simulink model "Cruise_Control_system_simulation"  (R2022b)
settings: Solver=VariableStepAuto  StartTime=0.0  StopTime=100  RelTol=1e-3
undefined symbols (not defined in the file): magnitude
libraries: slpidlib x5, simulink x1
settings Model: Creator=snazari  LastModifiedBy=ayush
settings SolverCC: ZeroCrossControl=DisableAll

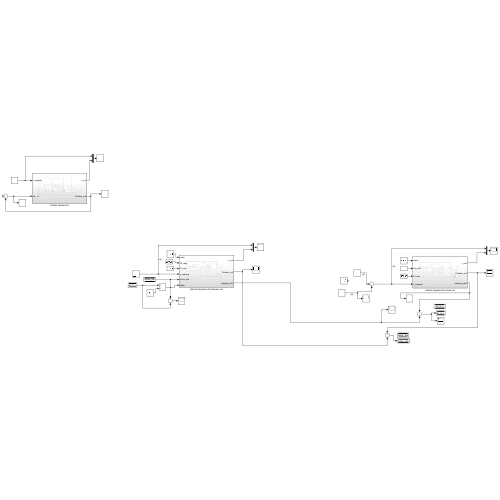
[thumbnail: Simulink's stored preview of the top-level diagram]
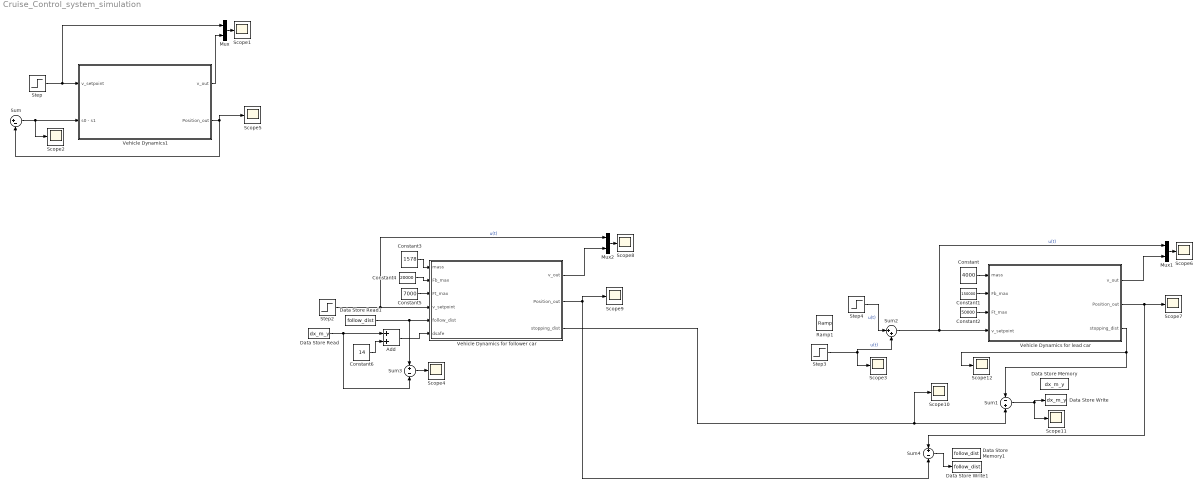
== system Cruise_Control_system_simulation ==
  Add : Sum
  Constant : Constant  Value=4000
  Constant1 : Constant  Value=150000
  Constant2 : Constant  Value=50000
  Constant3 : Constant  Value=1578
  Constant4 : Constant  Value=20000
  Constant5 : Constant  Value=7000
  Constant6 : Constant  Value=14
  Data Store Memory : DataStoreMemory  DataStoreName=dx_m_y  WriteAfterWriteMsg=warning  ShowAdditionalParam=off
  Data Store Memory1 : DataStoreMemory  DataStoreName=follow_dist  WriteAfterWriteMsg=warning  ShowAdditionalParam=off
  Data Store Read : DataStoreRead  DataStoreName=dx_m_y  IndexOptions=Index vector (dialog)  Indices=1  OutputSizes=1
  Data Store Read1 : DataStoreRead  DataStoreName=follow_dist  IndexOptions=Index vector (dialog)  Indices=1  OutputSizes=1
  Data Store Write : DataStoreWrite  DataStoreName=dx_m_y  IndexOptions=Index vector (dialog)  Indices=1  OutputSizes=1
  Data Store Write1 : DataStoreWrite  DataStoreName=follow_dist  IndexOptions=Index vector (dialog)  Indices=1  OutputSizes=1
  Mux : Mux  Inputs=2
  Mux1 : Mux  Inputs=2
  Mux2 : Mux  Inputs=2
  Ramp1 : simulink/Sources/Ramp  slope=-20  start=50  InitialOutput=0
  Scope{1..12} (12 alike) : Scope
  Step : Step  Before=3  After=35  SampleTime=0
  Step2 : Step  After=40  SampleTime=0
  Step3 : Step  Time=50  After=-35  SampleTime=0
  Step4 : Step  After=35  SampleTime=0
  Sum : Sum  Inputs=|+-
  Sum1 : Sum  Inputs=-+
  Sum2 : Sum  Inputs=|++
  Sum3 : Sum  Inputs=+-
  Sum4 : Sum  Inputs=+-
  Vehicle Dynamics for follower car : Subsystem
  Vehicle Dynamics for lead car : Subsystem
  Vehicle Dynamics1 : Subsystem
  wires:
  Constant1/1 -> Vehicle Dynamics for lead car/2(Fb_max)
  Constant/1 -> Vehicle Dynamics for lead car/1(mass)
  Sum2/1 -> Mux1/1, Vehicle Dynamics for lead car/4(v_setpoint)  "u(t)"
  Constant2/1 -> Vehicle Dynamics for lead car/3(Ft_max)
  Step3/1 -> Sum2/2, Scope3/1  "u(t)"
  Step4/1 -> Sum2/1  "u(t)"
  Mux1/1 -> Scope6/1
  Vehicle Dynamics for lead car/1(v_out) -> Mux1/2
  Vehicle Dynamics for lead car/2(Position_out) -> Sum4/1, Scope7/1
  Vehicle Dynamics for lead car/3(stopping_dist) -> Scope12/1, Sum1/1
  Step2/1 -> Mux2/1, Vehicle Dynamics for follower car/4(v_setpoint)  "u(t)"
  Mux2/1 -> Scope8/1
  Vehicle Dynamics for follower car/2(Position_out) -> Scope9/1, Sum4/2
  Constant3/1 -> Vehicle Dynamics for follower car/1(mass)
  Constant5/1 -> Vehicle Dynamics for follower car/3(Ft_max)
  Constant4/1 -> Vehicle Dynamics for follower car/2(Fb_max)
  Vehicle Dynamics for follower car/1(v_out) -> Mux2/2
  Vehicle Dynamics for follower car/3(stopping_dist) -> Scope10/1, Sum1/2
  Sum/1 -> Vehicle Dynamics1/2(s0 - s1), Scope2/1
  Vehicle Dynamics1/1(v_out) -> Mux/2
  Vehicle Dynamics1/2(Position_out) -> Scope5/1, Sum/2
  Mux/1 -> Scope1/1
  Step/1 -> Mux/1, Vehicle Dynamics1/1(v_setpoint)
  Sum4/1 -> Data Store Write1/1
  Data Store Read/1 -> Add/1, Sum3/2
  Data Store Read1/1 -> Vehicle Dynamics for follower car/5(follow_dist), Sum3/1
  Sum3/1 -> Scope4/1
  Constant6/1 -> Add/2
  Add/1 -> Vehicle Dynamics for follower car/6(dsafe)
  Sum1/1 -> Scope11/1, Data Store Write/1

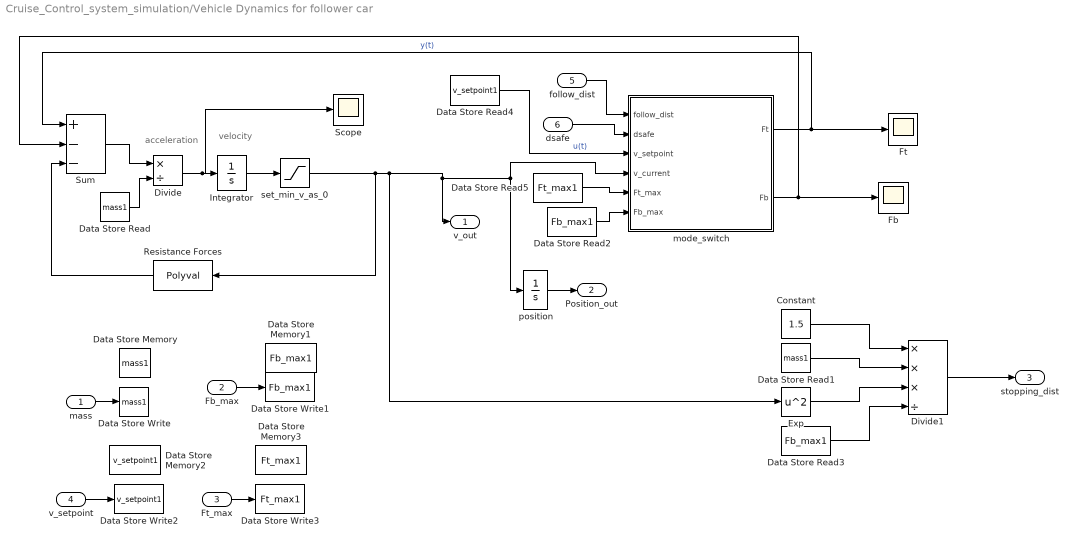
== system Cruise_Control_system_simulation/Vehicle Dynamics for follower car ==
  note: acceleration
  note: velocity
  mass : Inport
  Fb_max : Inport  Port=2
  Ft_max : Inport  Port=3
  v_setpoint : Inport  Port=4
  follow_dist : Inport  Port=5
  dsafe : Inport  Port=6
  Constant : Constant  Value=1.5
  Data Store Memory : DataStoreMemory  DataStoreName=mass1  WriteAfterWriteMsg=warning  ShowAdditionalParam=off
  Data Store Memory1 : DataStoreMemory  DataStoreName=Fb_max1  WriteAfterWriteMsg=warning  ShowAdditionalParam=off
  Data Store Memory2 : DataStoreMemory  DataStoreName=v_setpoint1  WriteAfterWriteMsg=warning  ShowAdditionalParam=off
  Data Store Memory3 : DataStoreMemory  DataStoreName=Ft_max1  WriteAfterWriteMsg=warning  ShowAdditionalParam=off
  Data Store Read : DataStoreRead  DataStoreName=mass1  IndexOptions=Index vector (dialog)  Indices=1  OutputSizes=1
  Data Store Read1 : DataStoreRead  DataStoreName=mass1  IndexOptions=Index vector (dialog)  Indices=1  OutputSizes=1
  Data Store Read2 : DataStoreRead  DataStoreName=Fb_max1  IndexOptions=Index vector (dialog)  Indices=1  OutputSizes=1
  Data Store Read3 : DataStoreRead  DataStoreName=Fb_max1  IndexOptions=Index vector (dialog)  Indices=1  OutputSizes=1
  Data Store Read4 : DataStoreRead  DataStoreName=v_setpoint1  IndexOptions=Index vector (dialog)  Indices=1  OutputSizes=1
  Data Store Read5 : DataStoreRead  DataStoreName=Ft_max1  IndexOptions=Index vector (dialog)  Indices=1  OutputSizes=1
  Data Store Write : DataStoreWrite  DataStoreName=mass1  IndexOptions=Index vector (dialog)  Indices=1  OutputSizes=1
  Data Store Write1 : DataStoreWrite  DataStoreName=Fb_max1  IndexOptions=Index vector (dialog)  Indices=1  OutputSizes=1
  Data Store Write2 : DataStoreWrite  DataStoreName=v_setpoint1  IndexOptions=Index vector (dialog)  Indices=1  OutputSizes=1
  Data Store Write3 : DataStoreWrite  DataStoreName=Ft_max1  IndexOptions=Index vector (dialog)  Indices=1  OutputSizes=1
  Divide : Product  Inputs=*/
  Divide1 : Product  Inputs=***/
  Exp : Math  Operator=square
  Fb : Scope
  Ft : Scope
  Integrator : Integrator
  Resistance Forces : Polyval  Coefs=[0.497 4.0349 97.33]
  Scope : Scope
  Sum : Sum  Inputs=+--
  mode_switch : Subsystem
  position : Integrator
  set_min_v_as_0 : Saturate  UpperLimit=3000  LowerLimit=0
  v_out : Outport
  Position_out : Outport  Port=2
  stopping_dist : Outport  Port=3
  wires:
  Data Store Read4/1 -> mode_switch/3(v_setpoint)  "u(t)"
  Integrator/1 -> set_min_v_as_0/1
  position/1 -> Position_out/1
  Resistance Forces/1 -> Sum/3
  Sum/1 -> Divide/1
  mass/1 -> Data Store Write/1
  Divide/1 -> Scope/1, Integrator/1
  mode_switch/1(Ft) -> Ft/1, Sum/1  "y(t)"
  mode_switch/2(Fb) -> Fb/1, Sum/2
  set_min_v_as_0/1 -> Exp/1, mode_switch/4(v_current), position/1, v_out/1, Resistance Forces/1
  Data Store Read5/1 -> mode_switch/5(Ft_max)
  Data Store Read2/1 -> mode_switch/6(Fb_max)
  Data Store Read/1 -> Divide/2
  Fb_max/1 -> Data Store Write1/1
  Constant/1 -> Divide1/1
  Data Store Read1/1 -> Divide1/2
  Exp/1 -> Divide1/3
  Data Store Read3/1 -> Divide1/4
  Divide1/1 -> stopping_dist/1
  v_setpoint/1 -> Data Store Write2/1
  Ft_max/1 -> Data Store Write3/1
  dsafe/1 -> mode_switch/2(dsafe)
  follow_dist/1 -> mode_switch/1(follow_dist)

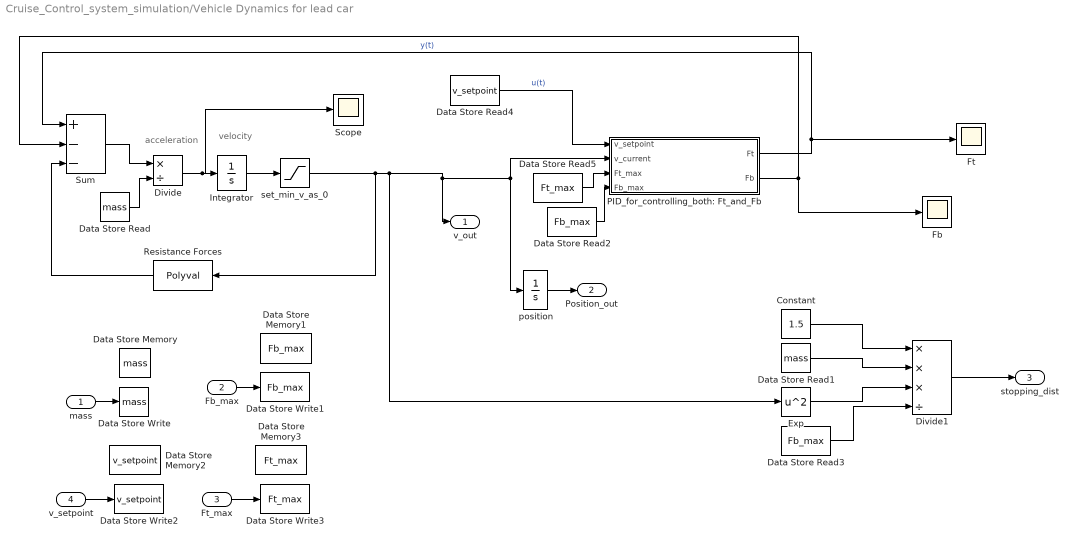
== system Cruise_Control_system_simulation/Vehicle Dynamics for lead car ==
  note: acceleration
  note: velocity
  mass : Inport
  Fb_max : Inport  Port=2
  Ft_max : Inport  Port=3
  v_setpoint : Inport  Port=4
  Constant : Constant  Value=1.5
  Data Store Memory : DataStoreMemory  DataStoreName=mass  WriteAfterWriteMsg=warning  ShowAdditionalParam=off
  Data Store Memory1 : DataStoreMemory  DataStoreName=Fb_max  WriteAfterWriteMsg=warning  ShowAdditionalParam=off
  Data Store Memory2 : DataStoreMemory  DataStoreName=v_setpoint  WriteAfterWriteMsg=warning  ShowAdditionalParam=off
  Data Store Memory3 : DataStoreMemory  DataStoreName=Ft_max  WriteAfterWriteMsg=warning  ShowAdditionalParam=off
  Data Store Read : DataStoreRead  DataStoreName=mass  IndexOptions=Index vector (dialog)  Indices=1  OutputSizes=1
  Data Store Read1 : DataStoreRead  DataStoreName=mass  IndexOptions=Index vector (dialog)  Indices=1  OutputSizes=1
  Data Store Read2 : DataStoreRead  DataStoreName=Fb_max  IndexOptions=Index vector (dialog)  Indices=1  OutputSizes=1
  Data Store Read3 : DataStoreRead  DataStoreName=Fb_max  IndexOptions=Index vector (dialog)  Indices=1  OutputSizes=1
  Data Store Read4 : DataStoreRead  DataStoreName=v_setpoint  IndexOptions=Index vector (dialog)  Indices=1  OutputSizes=1
  Data Store Read5 : DataStoreRead  DataStoreName=Ft_max  IndexOptions=Index vector (dialog)  Indices=1  OutputSizes=1
  Data Store Write : DataStoreWrite  DataStoreName=mass  IndexOptions=Index vector (dialog)  Indices=1  OutputSizes=1
  Data Store Write1 : DataStoreWrite  DataStoreName=Fb_max  IndexOptions=Index vector (dialog)  Indices=1  OutputSizes=1
  Data Store Write2 : DataStoreWrite  DataStoreName=v_setpoint  IndexOptions=Index vector (dialog)  Indices=1  OutputSizes=1
  Data Store Write3 : DataStoreWrite  DataStoreName=Ft_max  IndexOptions=Index vector (dialog)  Indices=1  OutputSizes=1
  Divide : Product  Inputs=*/
  Divide1 : Product  Inputs=***/
  Exp : Math  Operator=square
  Fb : Scope
  Ft : Scope
  Integrator : Integrator
  PID_for_controlling_both: Ft_and_Fb : Subsystem
  Resistance Forces : Polyval  Coefs=[0.497 4.0349 97.33]
  Scope : Scope
  Sum : Sum  Inputs=+--
  position : Integrator
  set_min_v_as_0 : Saturate  UpperLimit=3000  LowerLimit=0
  v_out : Outport
  Position_out : Outport  Port=2
  stopping_dist : Outport  Port=3
  wires:
  Data Store Read4/1 -> PID_for_controlling_both: Ft_and_Fb/1(v_setpoint)  "u(t)"
  Integrator/1 -> set_min_v_as_0/1
  position/1 -> Position_out/1
  Resistance Forces/1 -> Sum/3
  Sum/1 -> Divide/1
  mass/1 -> Data Store Write/1
  Divide/1 -> Scope/1, Integrator/1
  PID_for_controlling_both: Ft_and_Fb/1(Ft) -> Ft/1, Sum/1  "y(t)"
  PID_for_controlling_both: Ft_and_Fb/2(Fb) -> Fb/1, Sum/2
  set_min_v_as_0/1 -> Exp/1, PID_for_controlling_both: Ft_and_Fb/2(v_current), position/1, v_out/1, Resistance Forces/1
  Data Store Read5/1 -> PID_for_controlling_both: Ft_and_Fb/3(Ft_max)
  Data Store Read2/1 -> PID_for_controlling_both: Ft_and_Fb/4(Fb_max)
  Data Store Read/1 -> Divide/2
  Fb_max/1 -> Data Store Write1/1
  Constant/1 -> Divide1/1
  Data Store Read1/1 -> Divide1/2
  Exp/1 -> Divide1/3
  Divide1/1 -> stopping_dist/1
  v_setpoint/1 -> Data Store Write2/1
  Ft_max/1 -> Data Store Write3/1
  Data Store Read3/1 -> Divide1/4

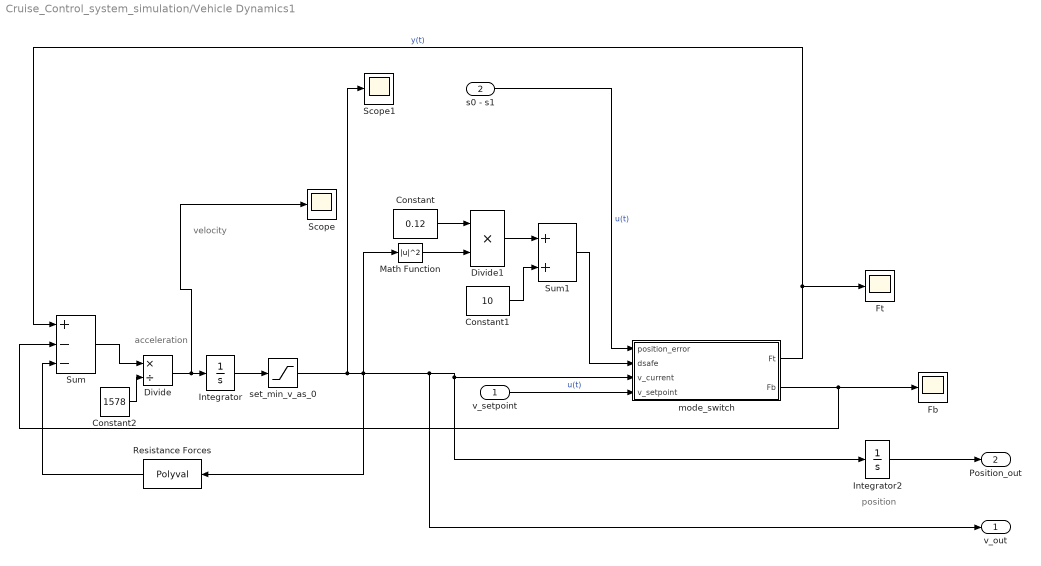
== system Cruise_Control_system_simulation/Vehicle Dynamics1 ==
  note: position
  note: acceleration
  note: velocity
  v_setpoint : Inport
  s0 - s1 : Inport  Port=2
  Constant : Constant  Value=0.12
  Constant1 : Constant  Value=10
  Constant2 : Constant  Value=1578
  Divide : Product  Inputs=*/
  Divide1 : Product  Inputs=**
  Fb : Scope
  Ft : Scope
  Integrator : Integrator
  Integrator2 : Integrator
  Math Function : Math  Operator=magnitude^2
  Resistance Forces : Polyval  Coefs=[0.497 4.0349 97.33]
  Scope : Scope
  Scope1 : Scope
  Sum : Sum  Inputs=+--
  Sum1 : Sum
  mode_switch : Subsystem
  set_min_v_as_0 : Saturate  UpperLimit=3000  LowerLimit=0
  v_out : Outport
  Position_out : Outport  Port=2
  wires:
  Divide/1 -> Scope/1, Integrator/1
  set_min_v_as_0/1 -> Math Function/1, mode_switch/3(v_current), Integrator2/1, v_out/1, Resistance Forces/1, Scope1/1
  Constant2/1 -> Divide/2
  mode_switch/2(Fb) -> Sum/2, Fb/1
  mode_switch/1(Ft) -> Sum/1, Ft/1  "y(t)"
  Resistance Forces/1 -> Sum/3
  Integrator2/1 -> Position_out/1
  Sum/1 -> Divide/1
  Integrator/1 -> set_min_v_as_0/1
  s0 - s1/1 -> mode_switch/1(position_error)  "u(t)"
  v_setpoint/1 -> mode_switch/4(v_setpoint)  "u(t)"
  Constant/1 -> Divide1/1
  Math Function/1 -> Divide1/2
  Divide1/1 -> Sum1/1
  Sum1/1 -> mode_switch/2(dsafe)
  Constant1/1 -> Sum1/2

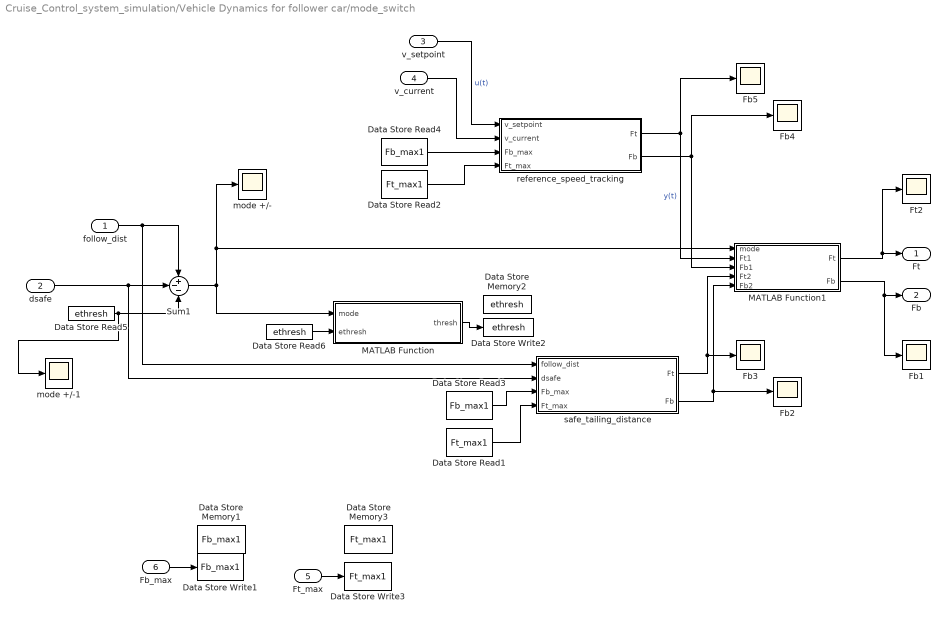
== system Cruise_Control_system_simulation/Vehicle Dynamics for follower car/mode_switch ==
  follow_dist : Inport
  dsafe : Inport  Port=2
  v_setpoint : Inport  Port=3
  v_current : Inport  Port=4
  Ft_max : Inport  Port=5
  Fb_max : Inport  Port=6
  Data Store Memory1 : DataStoreMemory  DataStoreName=Fb_max1  WriteAfterWriteMsg=warning  ShowAdditionalParam=off
  Data Store Memory2 : DataStoreMemory  DataStoreName=ethresh  WriteAfterWriteMsg=warning  ShowAdditionalParam=off
  Data Store Memory3 : DataStoreMemory  DataStoreName=Ft_max1  WriteAfterWriteMsg=warning  ShowAdditionalParam=off
  Data Store Read1 : DataStoreRead  DataStoreName=Ft_max1  IndexOptions=Index vector (dialog)  Indices=1  OutputSizes=1
  Data Store Read2 : DataStoreRead  DataStoreName=Ft_max1  IndexOptions=Index vector (dialog)  Indices=1  OutputSizes=1
  Data Store Read3 : DataStoreRead  DataStoreName=Fb_max1  IndexOptions=Index vector (dialog)  Indices=1  OutputSizes=1
  Data Store Read4 : DataStoreRead  DataStoreName=Fb_max1  IndexOptions=Index vector (dialog)  Indices=1  OutputSizes=1
  Data Store Read5 : DataStoreRead  DataStoreName=ethresh  IndexOptions=Index vector (dialog)  Indices=1  OutputSizes=1
  Data Store Read6 : DataStoreRead  DataStoreName=ethresh  IndexOptions=Index vector (dialog)  Indices=1  OutputSizes=1
  Data Store Write1 : DataStoreWrite  DataStoreName=Fb_max1  IndexOptions=Index vector (dialog)  Indices=1  OutputSizes=1
  Data Store Write2 : DataStoreWrite  DataStoreName=ethresh  IndexOptions=Index vector (dialog)  Indices=1  OutputSizes=1
  Data Store Write3 : DataStoreWrite  DataStoreName=Ft_max1  IndexOptions=Index vector (dialog)  Indices=1  OutputSizes=1
  Fb{1..5} (5 alike) : Scope
  Ft2 : Scope
  MATLAB Function : MATLAB Function  TreatAsAtomicUnit=on
  MATLAB Function1 : MATLAB Function  TreatAsAtomicUnit=on
  Sum1 : Sum  Inputs=+--
  mode +/- : Scope
  mode +/-1 : Scope
  reference_speed_tracking : Subsystem
  safe_tailing_distance : Subsystem
  Ft : Outport
  Fb : Outport  Port=2
  wires:
  dsafe/1 -> safe_tailing_distance/2(dsafe), Sum1/2
  v_setpoint/1 -> reference_speed_tracking/1(v_setpoint)  "u(t)"
  v_current/1 -> reference_speed_tracking/2(v_current)
  follow_dist/1 -> Sum1/1, safe_tailing_distance/1(follow_dist)
  MATLAB Function/1(thresh) -> Data Store Write2/1
  MATLAB Function1/1(Ft) -> Ft2/1, Ft/1
  MATLAB Function1/2(Fb) -> Fb1/1, Fb/1
  Sum1/1 -> MATLAB Function/1(mode), MATLAB Function1/1(mode), mode +/-/1
  reference_speed_tracking/1(Ft) -> Fb5/1, MATLAB Function1/2(Ft1)  "y(t)"
  safe_tailing_distance/1(Ft) -> Fb3/1, MATLAB Function1/4(Ft2)
  safe_tailing_distance/2(Fb) -> MATLAB Function1/5(Fb2), Fb2/1
  reference_speed_tracking/2(Fb) -> Fb4/1, MATLAB Function1/3(Fb1)
  Fb_max/1 -> Data Store Write1/1
  Ft_max/1 -> Data Store Write3/1
  Data Store Read3/1 -> safe_tailing_distance/3(Fb_max)
  Data Store Read1/1 -> safe_tailing_distance/4(Ft_max)
  Data Store Read4/1 -> reference_speed_tracking/3(Fb_max)
  Data Store Read2/1 -> reference_speed_tracking/4(Ft_max)
  Data Store Read5/1 -> mode +/-1/1, Sum1/3
  Data Store Read6/1 -> MATLAB Function/2(ethresh)

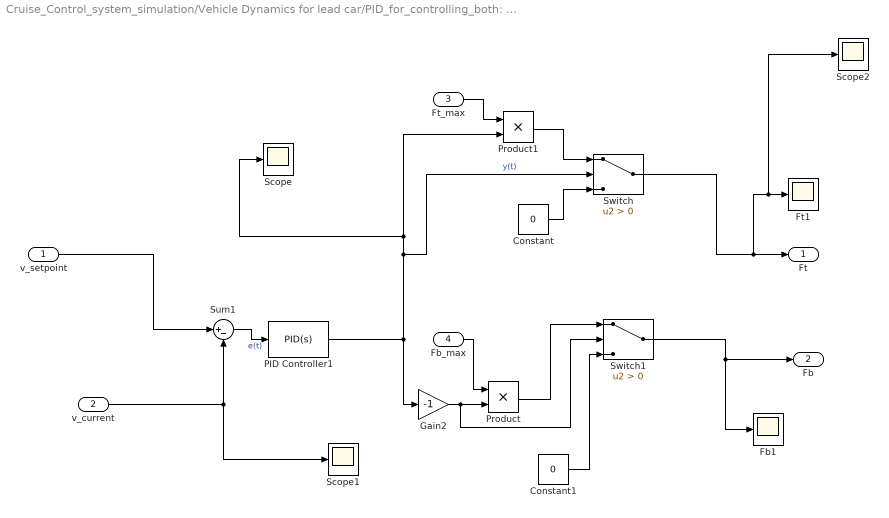
== system Cruise_Control_system_simulation/Vehicle Dynamics for lead car/PID_for_controlling_both: Ft_and_Fb ==
  v_setpoint : Inport
  v_current : Inport  Port=2
  Ft_max : Inport  Port=3
  Fb_max : Inport  Port=4
  Constant : Constant  Value=0
  Constant1 : Constant  Value=0
  Fb1 : Scope
  Ft1 : Scope
  Gain2 : Gain  Gain=-1
  PID Controller1 : slpidlib/PID Controller  Controller=PID  Form=Parallel  TimeDomain=Continuous-time  UseExternalTs=off  SampleTime=-1  IntegratorMethod=Forward Euler  FilterMethod=Forward Euler  ControllerParametersSource=internal  P=1  I=0.1  UseKiTs=off  D=0  N=100  UseFilter=on  TunerSelectOption=Transfer Function Based (PID Tuner App)  InitialConditionSource=internal  InitialConditionForIntegrator=0  InitialConditionForFilter=0  DifferentiatorICPrevScaledInput=0  ExternalReset=none  TrackingMode=off  Kt=1  LimitOutput=on  SatLimitsSource=internal  UpperSaturationLimit=1  LowerSaturationLimit=-1  LinearizeAsGain=on  AntiWindupMode=clamping  Kb=100  LimitIntegrator=off  UpperIntegratorSaturationLimit=inf  LowerIntegratorSaturationLimit=-inf  POutMin=[]  POutMax=[]  IOutMin=[]  IOutMax=[]  DOutMin=[]  DOutMax=[]  NOutMin=[]  NOutMax=[]  SumOutMin=[]  SumOutMax=[]  SaturationOutMin=[]  SaturationOutMax=[]  PParamMin=[]  PParamMax=[]  IParamMin=[]  IParamMax=[]  DParamMin=[]  DParamMax=[]  NParamMin=[]  NParamMax=[]  KbParamMin=[]  KbParamMax=[]  KtParamMin=[]  KtParamMax=[]  KbOutMin=[]  KbOutMax=[]  KtOutMin=[]  KtOutMax=[]  IntegratorOutMin=[]  IntegratorOutMax=[]  FilterOutMin=[]  FilterOutMax=[]  SumI1OutMin=[]  SumI1OutMax=[]  SumI2OutMin=[]  SumI2OutMax=[]  SumI3OutMin=[]  SumI3OutMax=[]  SumI4OutMin=[]  SumI4OutMax=[]  SumDOutMin=[]  SumDOutMax=[]  DifferentiatorOutMin=[]  DifferentiatorOutMax=[]  FilterDiffOutCoefMin=[]  FilterDiffOutCoefMax=[]  ReciprocalOutMin=[]  ReciprocalOutMax=[]  SumDenOutMin=[]  SumDenOutMax=[]  SumNumOutMin=[]  SumNumOutMax=[]  DivideOutMin=[]  DivideOutMax=[]  UdiffTsProdOutMin=[]  UdiffTsProdOutMax=[]  NTsProdOutMin=[]  NTsProdOutMax=[]  UintegralTsProdOutMin=[]  UintegralTsProdOutMax=[]  UngainTsProdOutMin=[]  UngainTsProdOutMax=[]  ClampingZeroOutDataTypeStr=Inherit: Inherit via back propagation  ClampingZeroOutMin=[]  ClampingZeroOutMax=[]  FilterDenConstantOutDataTypeStr=Inherit: Inherit via back propagation  FilterDenConstantOutMin=[]  FilterDenConstantOutMax=[]  PCopyOutDataTypeStr=Inherit: Inherit via back propagation  PCopyOutMin=[]  PCopyOutMax=[]  NCopyOutDataTypeStr=Inherit: Inherit via back propagation  NCopyOutMin=[]  NCopyOutMax=[]  IntegratorContinuousStateAttributes=''  IntegratorStateMustResolveToSignalObject=off  IntegratorRTWStateStorageClass=Auto  FilterContinuousStateAttributes=''  FilterStateMustResolveToSignalObject=off  FilterRTWStateStorageClass=Auto  ParallelPVariant=InternalParameters  IdealPVariant=Disabled  IVariant=InternalParameters  DVariant=InternalParameters  IntegratorVariant=Continuous  SatVariant=Enabled  AWVariant=ContClampingParallel  PCopyVariant=Disabled  TRVariant=Disabled  FdbkBlocksVariant=Forward  IdealPFdbkVariant=Disabled  SatFdbkVariant=Disabled  DerivativeFilterVariant=ContFilter  NVariant=InternalParameters  NCopyVariant=Disabled  FilterICVariant=InternalICsFilter  IntegratorICVariant=InternalICs  ExternalResetVariant=Disabled  TRSumVariant=Passthrough  SumFdbkVariant=Disabled  SumVariant=Sum_PID  TsampFilterVariant=InternalTs  TsampNgainVariant=Passthrough  TsampIntegralVariant=Passthrough  ExternalSaturationOutDataTypeStr=Inherit: Same as second input
  Product : Product
  Product1 : Product
  Scope : Scope
  Scope1 : Scope
  Scope2 : Scope
  Sum1 : Sum  Inputs=|+-
  Switch : Switch  Criteria=u2 > Threshold  SaturateOnIntegerOverflow=off  InputSameDT=off
  Switch1 : Switch  Criteria=u2 > Threshold  SaturateOnIntegerOverflow=off  InputSameDT=off
  Ft : Outport
  Fb : Outport  Port=2
  wires:
  v_setpoint/1 -> Sum1/1
  PID Controller1/1 -> Product1/2, Scope/1, Switch/2, Gain2/1  "y(t)"
  Sum1/1 -> PID Controller1/1  "e(t)"
  v_current/1 -> Scope1/1, Sum1/2
  Switch1/1 -> Fb1/1, Fb/1
  Switch/1 -> Scope2/1, Ft1/1, Ft/1
  Product1/1 -> Switch/1
  Constant/1 -> Switch/3
  Constant1/1 -> Switch1/3
  Product/1 -> Switch1/1
  Gain2/1 -> Switch1/2, Product/2
  Fb_max/1 -> Product/1
  Ft_max/1 -> Product1/1

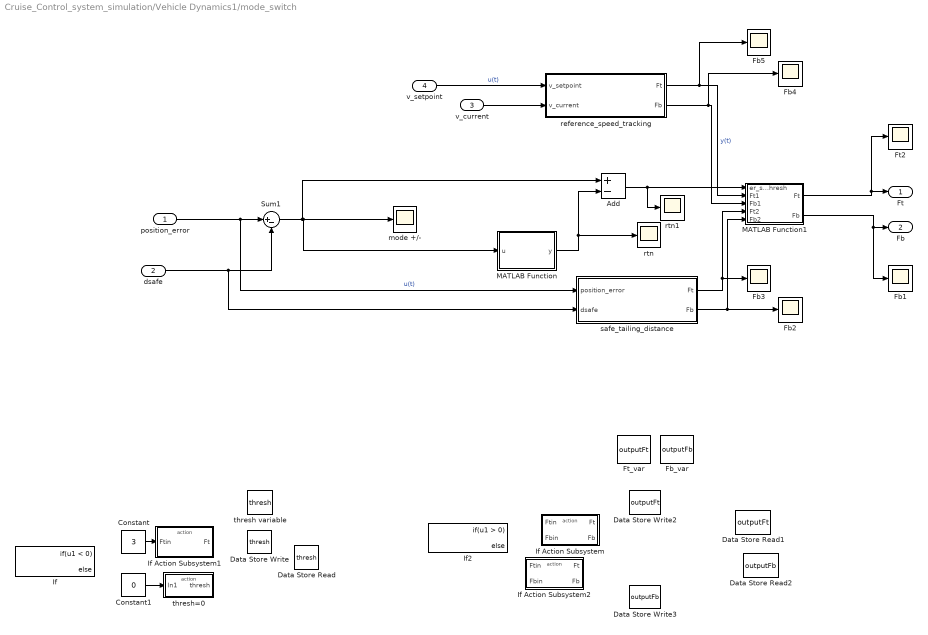
== system Cruise_Control_system_simulation/Vehicle Dynamics1/mode_switch ==
  position_error : Inport
  dsafe : Inport  Port=2
  v_current : Inport  Port=3
  v_setpoint : Inport  Port=4
  Add : Sum  Inputs=+-
  Constant : Constant  Value=3
  Constant1 : Constant  Value=0
  Data Store Read : DataStoreRead  DataStoreName=thresh  IndexOptions=Index vector (dialog)  Indices=1  OutputSizes=1
  Data Store Read1 : DataStoreRead  DataStoreName=outputFt  IndexOptions=Index vector (dialog)  Indices=1  OutputSizes=1
  Data Store Read2 : DataStoreRead  DataStoreName=outputFb  IndexOptions=Index vector (dialog)  Indices=1  OutputSizes=1
  Data Store Write : DataStoreWrite  DataStoreName=thresh  IndexOptions=Index vector (dialog)  Indices=1  OutputSizes=1
  Data Store Write2 : DataStoreWrite  DataStoreName=outputFt  IndexOptions=Index vector (dialog)  Indices=1  OutputSizes=1
  Data Store Write3 : DataStoreWrite  DataStoreName=outputFb  IndexOptions=Index vector (dialog)  Indices=1  OutputSizes=1
  Fb{1..5} (5 alike) : Scope
  Fb_var : DataStoreMemory  DataStoreName=outputFb  WriteAfterWriteMsg=warning  ShowAdditionalParam=off
  Ft2 : Scope
  Ft_var : DataStoreMemory  DataStoreName=outputFt  WriteAfterWriteMsg=warning  ShowAdditionalParam=off
  If : If  IfExpression=u1 < 0
  If Action Subsystem : Subsystem  TreatAsAtomicUnit=on
  If Action Subsystem1 : Subsystem  TreatAsAtomicUnit=on
  If Action Subsystem2 : Subsystem  TreatAsAtomicUnit=on
  If2 : If
  MATLAB Function : MATLAB Function  TreatAsAtomicUnit=on
  MATLAB Function1 : MATLAB Function  TreatAsAtomicUnit=on
  Sum1 : Sum  Inputs=|+-
  mode +/- : Scope
  reference_speed_tracking : Subsystem
  rtn : Scope
  rtn1 : Scope
  safe_tailing_distance : Subsystem
  thresh variable : DataStoreMemory  DataStoreName=thresh  WriteAfterWriteMsg=warning  ShowAdditionalParam=off
  thresh=0 : Subsystem  TreatAsAtomicUnit=on
  Ft : Outport
  Fb : Outport  Port=2
  wires:
  dsafe/1 -> safe_tailing_distance/2(dsafe), Sum1/2
  v_setpoint/1 -> reference_speed_tracking/1(v_setpoint)  "u(t)"
  v_current/1 -> reference_speed_tracking/2(v_current)
  position_error/1 -> safe_tailing_distance/1(position_error), Sum1/1  "u(t)"
  MATLAB Function/1(y) -> Add/2, rtn/1
  Add/1 -> rtn1/1, MATLAB Function1/1(er_sub_thresh)
  MATLAB Function1/1(Ft) -> Ft2/1, Ft/1
  MATLAB Function1/2(Fb) -> Fb1/1, Fb/1
  Constant/1 -> If Action Subsystem1/1(Ftin)
  Constant1/1 -> thresh=0/1(In1)
  Sum1/1 -> Add/1, MATLAB Function/1(u), mode +/-/1
  reference_speed_tracking/1(Ft) -> Fb5/1, MATLAB Function1/2(Ft1)  "y(t)"
  safe_tailing_distance/1(Ft) -> Fb3/1, MATLAB Function1/4(Ft2)
  safe_tailing_distance/2(Fb) -> MATLAB Function1/5(Fb2), Fb2/1
  reference_speed_tracking/2(Fb) -> Fb4/1, MATLAB Function1/3(Fb1)

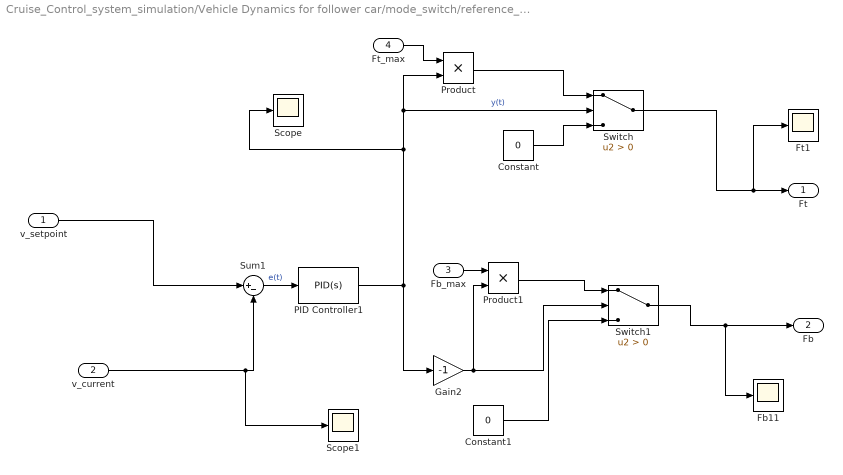
== system Cruise_Control_system_simulation/Vehicle Dynamics for follower car/mode_switch/reference_speed_tracking ==
  v_setpoint : Inport
  v_current : Inport  Port=2
  Fb_max : Inport  Port=3
  Ft_max : Inport  Port=4
  Constant : Constant  Value=0
  Constant1 : Constant  Value=0
  Fb11 : Scope
  Ft1 : Scope
  Gain2 : Gain  Gain=-1
  PID Controller1 : slpidlib/PID Controller  Controller=PID  Form=Parallel  TimeDomain=Continuous-time  UseExternalTs=off  SampleTime=-1  IntegratorMethod=Forward Euler  FilterMethod=Forward Euler  ControllerParametersSource=internal  P=1  I=0.1  UseKiTs=off  D=0  N=100  UseFilter=on  TunerSelectOption=Transfer Function Based (PID Tuner App)  InitialConditionSource=internal  InitialConditionForIntegrator=0  InitialConditionForFilter=0  DifferentiatorICPrevScaledInput=0  ExternalReset=none  TrackingMode=off  Kt=1  LimitOutput=on  SatLimitsSource=internal  UpperSaturationLimit=1  LowerSaturationLimit=-1  LinearizeAsGain=on  AntiWindupMode=clamping  Kb=100  LimitIntegrator=off  UpperIntegratorSaturationLimit=inf  LowerIntegratorSaturationLimit=-inf  POutMin=[]  POutMax=[]  IOutMin=[]  IOutMax=[]  DOutMin=[]  DOutMax=[]  NOutMin=[]  NOutMax=[]  SumOutMin=[]  SumOutMax=[]  SaturationOutMin=[]  SaturationOutMax=[]  PParamMin=[]  PParamMax=[]  IParamMin=[]  IParamMax=[]  DParamMin=[]  DParamMax=[]  NParamMin=[]  NParamMax=[]  KbParamMin=[]  KbParamMax=[]  KtParamMin=[]  KtParamMax=[]  KbOutMin=[]  KbOutMax=[]  KtOutMin=[]  KtOutMax=[]  IntegratorOutMin=[]  IntegratorOutMax=[]  FilterOutMin=[]  FilterOutMax=[]  SumI1OutMin=[]  SumI1OutMax=[]  SumI2OutMin=[]  SumI2OutMax=[]  SumI3OutMin=[]  SumI3OutMax=[]  SumI4OutMin=[]  SumI4OutMax=[]  SumDOutMin=[]  SumDOutMax=[]  DifferentiatorOutMin=[]  DifferentiatorOutMax=[]  FilterDiffOutCoefMin=[]  FilterDiffOutCoefMax=[]  ReciprocalOutMin=[]  ReciprocalOutMax=[]  SumDenOutMin=[]  SumDenOutMax=[]  SumNumOutMin=[]  SumNumOutMax=[]  DivideOutMin=[]  DivideOutMax=[]  UdiffTsProdOutMin=[]  UdiffTsProdOutMax=[]  NTsProdOutMin=[]  NTsProdOutMax=[]  UintegralTsProdOutMin=[]  UintegralTsProdOutMax=[]  UngainTsProdOutMin=[]  UngainTsProdOutMax=[]  ClampingZeroOutDataTypeStr=Inherit: Inherit via back propagation  ClampingZeroOutMin=[]  ClampingZeroOutMax=[]  FilterDenConstantOutDataTypeStr=Inherit: Inherit via back propagation  FilterDenConstantOutMin=[]  FilterDenConstantOutMax=[]  PCopyOutDataTypeStr=Inherit: Inherit via back propagation  PCopyOutMin=[]  PCopyOutMax=[]  NCopyOutDataTypeStr=Inherit: Inherit via back propagation  NCopyOutMin=[]  NCopyOutMax=[]  IntegratorContinuousStateAttributes=''  IntegratorStateMustResolveToSignalObject=off  IntegratorRTWStateStorageClass=Auto  FilterContinuousStateAttributes=''  FilterStateMustResolveToSignalObject=off  FilterRTWStateStorageClass=Auto  ParallelPVariant=InternalParameters  IdealPVariant=Disabled  IVariant=InternalParameters  DVariant=InternalParameters  IntegratorVariant=Continuous  SatVariant=Enabled  AWVariant=ContClampingParallel  PCopyVariant=Disabled  TRVariant=Disabled  FdbkBlocksVariant=Forward  IdealPFdbkVariant=Disabled  SatFdbkVariant=Disabled  DerivativeFilterVariant=ContFilter  NVariant=InternalParameters  NCopyVariant=Disabled  FilterICVariant=InternalICsFilter  IntegratorICVariant=InternalICs  ExternalResetVariant=Disabled  TRSumVariant=Passthrough  SumFdbkVariant=Disabled  SumVariant=Sum_PID  TsampFilterVariant=InternalTs  TsampNgainVariant=Passthrough  TsampIntegralVariant=Passthrough  ExternalSaturationOutDataTypeStr=Inherit: Same as second input
  Product : Product
  Product1 : Product
  Scope : Scope
  Scope1 : Scope
  Sum1 : Sum  Inputs=|+-
  Switch : Switch  Criteria=u2 > Threshold  SaturateOnIntegerOverflow=off  InputSameDT=off
  Switch1 : Switch  Criteria=u2 > Threshold  SaturateOnIntegerOverflow=off  InputSameDT=off
  Ft : Outport
  Fb : Outport  Port=2
  wires:
  v_setpoint/1 -> Sum1/1
  PID Controller1/1 -> Gain2/1, Switch/2, Product/2, Scope/1  "y(t)"
  Sum1/1 -> PID Controller1/1  "e(t)"
  v_current/1 -> Scope1/1, Sum1/2
  Switch1/1 -> Fb11/1, Fb/1
  Switch/1 -> Ft/1, Ft1/1
  Product/1 -> Switch/1
  Constant/1 -> Switch/3
  Constant1/1 -> Switch1/3
  Gain2/1 -> Product1/2, Switch1/2
  Ft_max/1 -> Product/1
  Fb_max/1 -> Product1/1
  Product1/1 -> Switch1/1

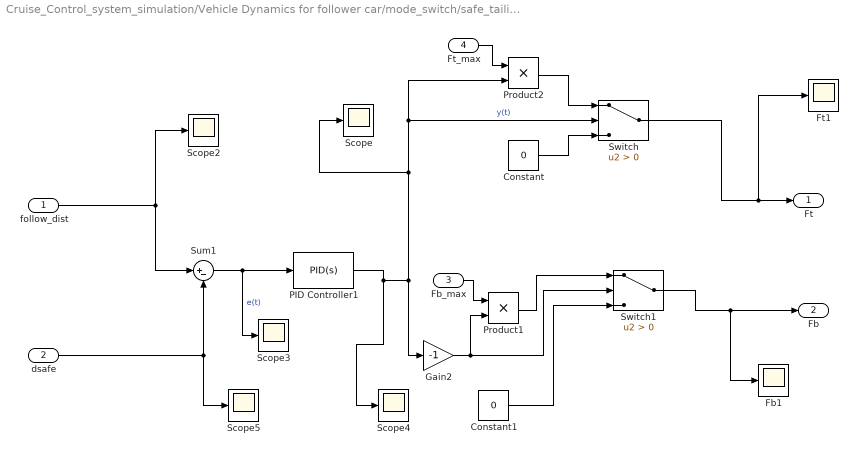
== system Cruise_Control_system_simulation/Vehicle Dynamics for follower car/mode_switch/safe_tailing_distance ==
  follow_dist : Inport
  dsafe : Inport  Port=2
  Fb_max : Inport  Port=3
  Ft_max : Inport  Port=4
  Constant : Constant  Value=0
  Constant1 : Constant  Value=0
  Fb1 : Scope
  Ft1 : Scope
  Gain2 : Gain  Gain=-1
  PID Controller1 : slpidlib/PID Controller  Controller=PID  Form=Parallel  TimeDomain=Continuous-time  UseExternalTs=off  SampleTime=-1  IntegratorMethod=Forward Euler  FilterMethod=Forward Euler  ControllerParametersSource=internal  P=0.2  I=0.1  UseKiTs=off  D=0  N=100  UseFilter=on  TunerSelectOption=Transfer Function Based (PID Tuner App)  InitialConditionSource=internal  InitialConditionForIntegrator=0  InitialConditionForFilter=0  DifferentiatorICPrevScaledInput=0  ExternalReset=none  TrackingMode=off  Kt=1  LimitOutput=on  SatLimitsSource=internal  UpperSaturationLimit=1  LowerSaturationLimit=-1  LinearizeAsGain=on  AntiWindupMode=clamping  Kb=100  LimitIntegrator=off  UpperIntegratorSaturationLimit=inf  LowerIntegratorSaturationLimit=-inf  POutMin=[]  POutMax=[]  IOutMin=[]  IOutMax=[]  DOutMin=[]  DOutMax=[]  NOutMin=[]  NOutMax=[]  SumOutMin=[]  SumOutMax=[]  SaturationOutMin=[]  SaturationOutMax=[]  PParamMin=[]  PParamMax=[]  IParamMin=[]  IParamMax=[]  DParamMin=[]  DParamMax=[]  NParamMin=[]  NParamMax=[]  KbParamMin=[]  KbParamMax=[]  KtParamMin=[]  KtParamMax=[]  KbOutMin=[]  KbOutMax=[]  KtOutMin=[]  KtOutMax=[]  IntegratorOutMin=[]  IntegratorOutMax=[]  FilterOutMin=[]  FilterOutMax=[]  SumI1OutMin=[]  SumI1OutMax=[]  SumI2OutMin=[]  SumI2OutMax=[]  SumI3OutMin=[]  SumI3OutMax=[]  SumI4OutMin=[]  SumI4OutMax=[]  SumDOutMin=[]  SumDOutMax=[]  DifferentiatorOutMin=[]  DifferentiatorOutMax=[]  FilterDiffOutCoefMin=[]  FilterDiffOutCoefMax=[]  ReciprocalOutMin=[]  ReciprocalOutMax=[]  SumDenOutMin=[]  SumDenOutMax=[]  SumNumOutMin=[]  SumNumOutMax=[]  DivideOutMin=[]  DivideOutMax=[]  UdiffTsProdOutMin=[]  UdiffTsProdOutMax=[]  NTsProdOutMin=[]  NTsProdOutMax=[]  UintegralTsProdOutMin=[]  UintegralTsProdOutMax=[]  UngainTsProdOutMin=[]  UngainTsProdOutMax=[]  ClampingZeroOutDataTypeStr=Inherit: Inherit via back propagation  ClampingZeroOutMin=[]  ClampingZeroOutMax=[]  FilterDenConstantOutDataTypeStr=Inherit: Inherit via back propagation  FilterDenConstantOutMin=[]  FilterDenConstantOutMax=[]  PCopyOutDataTypeStr=Inherit: Inherit via back propagation  PCopyOutMin=[]  PCopyOutMax=[]  NCopyOutDataTypeStr=Inherit: Inherit via back propagation  NCopyOutMin=[]  NCopyOutMax=[]  IntegratorContinuousStateAttributes=''  IntegratorStateMustResolveToSignalObject=off  IntegratorRTWStateStorageClass=Auto  FilterContinuousStateAttributes=''  FilterStateMustResolveToSignalObject=off  FilterRTWStateStorageClass=Auto  ParallelPVariant=InternalParameters  IdealPVariant=Disabled  IVariant=InternalParameters  DVariant=InternalParameters  IntegratorVariant=Continuous  SatVariant=Enabled  AWVariant=ContClampingParallel  PCopyVariant=Disabled  TRVariant=Disabled  FdbkBlocksVariant=Forward  IdealPFdbkVariant=Disabled  SatFdbkVariant=Disabled  DerivativeFilterVariant=ContFilter  NVariant=InternalParameters  NCopyVariant=Disabled  FilterICVariant=InternalICsFilter  IntegratorICVariant=InternalICs  ExternalResetVariant=Disabled  TRSumVariant=Passthrough  SumFdbkVariant=Disabled  SumVariant=Sum_PID  TsampFilterVariant=InternalTs  TsampNgainVariant=Passthrough  TsampIntegralVariant=Passthrough  ExternalSaturationOutDataTypeStr=Inherit: Same as second input
  Product1 : Product
  Product2 : Product
  Scope{,2..5} (5 alike) : Scope
  Sum1 : Sum  Inputs=|+-
  Switch : Switch  Criteria=u2 > Threshold  SaturateOnIntegerOverflow=off  InputSameDT=off
  Switch1 : Switch  Criteria=u2 > Threshold  SaturateOnIntegerOverflow=off  InputSameDT=off
  Ft : Outport
  Fb : Outport  Port=2
  wires:
  Gain2/1 -> Product1/2, Switch1/2
  Constant1/1 -> Switch1/3
  PID Controller1/1 -> Scope4/1, Switch/2, Product2/2, Scope/1, Gain2/1  "y(t)"
  Constant/1 -> Switch/3
  Product1/1 -> Switch1/1
  follow_dist/1 -> Scope2/1, Sum1/1
  Product2/1 -> Switch/1
  Switch/1 -> Ft1/1, Ft/1
  Switch1/1 -> Fb1/1, Fb/1
  dsafe/1 -> Scope5/1, Sum1/2
  Sum1/1 -> Scope3/1, PID Controller1/1  "e(t)"
  Fb_max/1 -> Product1/1
  Ft_max/1 -> Product2/1

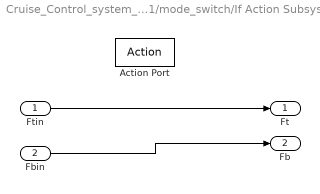
== system Cruise_Control_system_simulation/Vehicle Dynamics1/mode_switch/If Action Subsystem ==
  Ftin : Inport
  Fbin : Inport  Port=2
  Action Port : ActionPort
  Ft : Outport
  Fb : Outport  Port=2
  wires:
  Ftin/1 -> Ft/1
  Fbin/1 -> Fb/1

== system Cruise_Control_system_simulation/Vehicle Dynamics1/mode_switch/If Action Subsystem1 ==
  Ftin : Inport
  Action Port : ActionPort
  Ft : Outport
  wires:
  Ftin/1 -> Ft/1

== system Cruise_Control_system_simulation/Vehicle Dynamics1/mode_switch/If Action Subsystem2 ==
  Ftin : Inport
  Fbin : Inport  Port=2
  Action Port : ActionPort
  Ft : Outport
  Fb : Outport  Port=2
  wires:
  Ftin/1 -> Ft/1
  Fbin/1 -> Fb/1

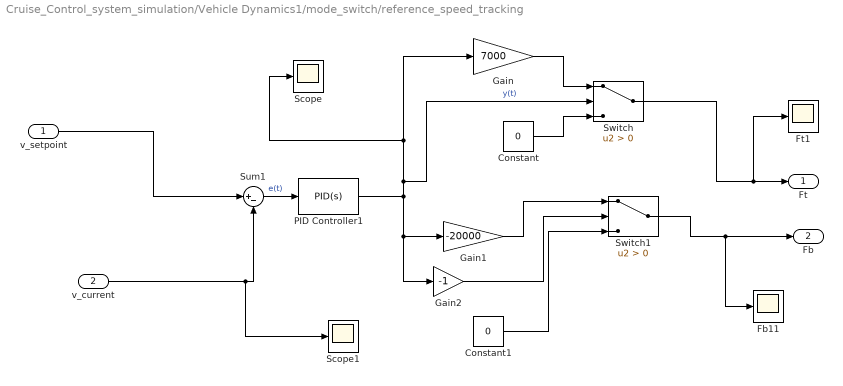
== system Cruise_Control_system_simulation/Vehicle Dynamics1/mode_switch/reference_speed_tracking ==
  v_setpoint : Inport
  v_current : Inport  Port=2
  Constant : Constant  Value=0
  Constant1 : Constant  Value=0
  Fb11 : Scope
  Ft1 : Scope
  Gain : Gain  Gain=7000
  Gain1 : Gain  Gain=-20000
  Gain2 : Gain  Gain=-1
  PID Controller1 : slpidlib/PID Controller  Controller=PID  Form=Parallel  TimeDomain=Continuous-time  UseExternalTs=off  SampleTime=-1  IntegratorMethod=Forward Euler  FilterMethod=Forward Euler  ControllerParametersSource=internal  P=1  I=0.1  UseKiTs=off  D=0  N=100  UseFilter=on  TunerSelectOption=Transfer Function Based (PID Tuner App)  InitialConditionSource=internal  InitialConditionForIntegrator=0  InitialConditionForFilter=0  DifferentiatorICPrevScaledInput=0  ExternalReset=none  TrackingMode=off  Kt=1  LimitOutput=on  SatLimitsSource=internal  UpperSaturationLimit=1  LowerSaturationLimit=-1  LinearizeAsGain=on  AntiWindupMode=clamping  Kb=100  LimitIntegrator=off  UpperIntegratorSaturationLimit=inf  LowerIntegratorSaturationLimit=-inf  POutMin=[]  POutMax=[]  IOutMin=[]  IOutMax=[]  DOutMin=[]  DOutMax=[]  NOutMin=[]  NOutMax=[]  SumOutMin=[]  SumOutMax=[]  SaturationOutMin=[]  SaturationOutMax=[]  PParamMin=[]  PParamMax=[]  IParamMin=[]  IParamMax=[]  DParamMin=[]  DParamMax=[]  NParamMin=[]  NParamMax=[]  KbParamMin=[]  KbParamMax=[]  KtParamMin=[]  KtParamMax=[]  KbOutMin=[]  KbOutMax=[]  KtOutMin=[]  KtOutMax=[]  IntegratorOutMin=[]  IntegratorOutMax=[]  FilterOutMin=[]  FilterOutMax=[]  SumI1OutMin=[]  SumI1OutMax=[]  SumI2OutMin=[]  SumI2OutMax=[]  SumI3OutMin=[]  SumI3OutMax=[]  SumI4OutMin=[]  SumI4OutMax=[]  SumDOutMin=[]  SumDOutMax=[]  DifferentiatorOutMin=[]  DifferentiatorOutMax=[]  FilterDiffOutCoefMin=[]  FilterDiffOutCoefMax=[]  ReciprocalOutMin=[]  ReciprocalOutMax=[]  SumDenOutMin=[]  SumDenOutMax=[]  SumNumOutMin=[]  SumNumOutMax=[]  DivideOutMin=[]  DivideOutMax=[]  UdiffTsProdOutMin=[]  UdiffTsProdOutMax=[]  NTsProdOutMin=[]  NTsProdOutMax=[]  UintegralTsProdOutMin=[]  UintegralTsProdOutMax=[]  UngainTsProdOutMin=[]  UngainTsProdOutMax=[]  ClampingZeroOutDataTypeStr=Inherit: Inherit via back propagation  ClampingZeroOutMin=[]  ClampingZeroOutMax=[]  FilterDenConstantOutDataTypeStr=Inherit: Inherit via back propagation  FilterDenConstantOutMin=[]  FilterDenConstantOutMax=[]  PCopyOutDataTypeStr=Inherit: Inherit via back propagation  PCopyOutMin=[]  PCopyOutMax=[]  NCopyOutDataTypeStr=Inherit: Inherit via back propagation  NCopyOutMin=[]  NCopyOutMax=[]  IntegratorContinuousStateAttributes=''  IntegratorStateMustResolveToSignalObject=off  IntegratorRTWStateStorageClass=Auto  FilterContinuousStateAttributes=''  FilterStateMustResolveToSignalObject=off  FilterRTWStateStorageClass=Auto  ParallelPVariant=InternalParameters  IdealPVariant=Disabled  IVariant=InternalParameters  DVariant=InternalParameters  IntegratorVariant=Continuous  SatVariant=Enabled  AWVariant=ContClampingParallel  PCopyVariant=Disabled  TRVariant=Disabled  FdbkBlocksVariant=Forward  IdealPFdbkVariant=Disabled  SatFdbkVariant=Disabled  DerivativeFilterVariant=ContFilter  NVariant=InternalParameters  NCopyVariant=Disabled  FilterICVariant=InternalICsFilter  IntegratorICVariant=InternalICs  ExternalResetVariant=Disabled  TRSumVariant=Passthrough  SumFdbkVariant=Disabled  SumVariant=Sum_PID  TsampFilterVariant=InternalTs  TsampNgainVariant=Passthrough  TsampIntegralVariant=Passthrough  ExternalSaturationOutDataTypeStr=Inherit: Same as second input
  Scope : Scope
  Scope1 : Scope
  Sum1 : Sum  Inputs=|+-
  Switch : Switch  Criteria=u2 > Threshold  SaturateOnIntegerOverflow=off  InputSameDT=off
  Switch1 : Switch  Criteria=u2 > Threshold  SaturateOnIntegerOverflow=off  InputSameDT=off
  Ft : Outport
  Fb : Outport  Port=2
  wires:
  v_setpoint/1 -> Sum1/1
  PID Controller1/1 -> Gain2/1, Gain1/1, Scope/1, Gain/1, Switch/2  "y(t)"
  Sum1/1 -> PID Controller1/1  "e(t)"
  v_current/1 -> Scope1/1, Sum1/2
  Switch1/1 -> Fb11/1, Fb/1
  Switch/1 -> Ft/1, Ft1/1
  Gain/1 -> Switch/1
  Constant/1 -> Switch/3
  Gain1/1 -> Switch1/1
  Constant1/1 -> Switch1/3
  Gain2/1 -> Switch1/2

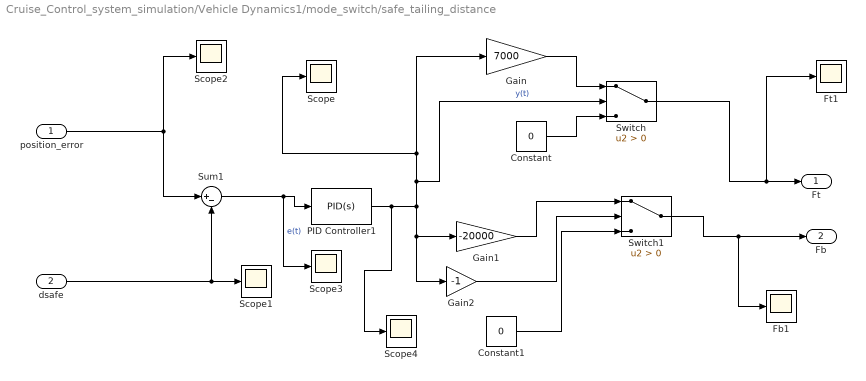
== system Cruise_Control_system_simulation/Vehicle Dynamics1/mode_switch/safe_tailing_distance ==
  position_error : Inport
  dsafe : Inport  Port=2
  Constant : Constant  Value=0
  Constant1 : Constant  Value=0
  Fb1 : Scope
  Ft1 : Scope
  Gain : Gain  Gain=7000
  Gain1 : Gain  Gain=-20000
  Gain2 : Gain  Gain=-1
  PID Controller1 : slpidlib/PID Controller  Controller=PID  Form=Parallel  TimeDomain=Continuous-time  UseExternalTs=off  SampleTime=-1  IntegratorMethod=Forward Euler  FilterMethod=Forward Euler  ControllerParametersSource=internal  P=1  I=0.1  UseKiTs=off  D=0  N=100  UseFilter=on  TunerSelectOption=Transfer Function Based (PID Tuner App)  InitialConditionSource=internal  InitialConditionForIntegrator=0  InitialConditionForFilter=0  DifferentiatorICPrevScaledInput=0  ExternalReset=none  TrackingMode=off  Kt=1  LimitOutput=on  SatLimitsSource=internal  UpperSaturationLimit=1  LowerSaturationLimit=-1  LinearizeAsGain=on  AntiWindupMode=clamping  Kb=100  LimitIntegrator=off  UpperIntegratorSaturationLimit=inf  LowerIntegratorSaturationLimit=-inf  POutMin=[]  POutMax=[]  IOutMin=[]  IOutMax=[]  DOutMin=[]  DOutMax=[]  NOutMin=[]  NOutMax=[]  SumOutMin=[]  SumOutMax=[]  SaturationOutMin=[]  SaturationOutMax=[]  PParamMin=[]  PParamMax=[]  IParamMin=[]  IParamMax=[]  DParamMin=[]  DParamMax=[]  NParamMin=[]  NParamMax=[]  KbParamMin=[]  KbParamMax=[]  KtParamMin=[]  KtParamMax=[]  KbOutMin=[]  KbOutMax=[]  KtOutMin=[]  KtOutMax=[]  IntegratorOutMin=[]  IntegratorOutMax=[]  FilterOutMin=[]  FilterOutMax=[]  SumI1OutMin=[]  SumI1OutMax=[]  SumI2OutMin=[]  SumI2OutMax=[]  SumI3OutMin=[]  SumI3OutMax=[]  SumI4OutMin=[]  SumI4OutMax=[]  SumDOutMin=[]  SumDOutMax=[]  DifferentiatorOutMin=[]  DifferentiatorOutMax=[]  FilterDiffOutCoefMin=[]  FilterDiffOutCoefMax=[]  ReciprocalOutMin=[]  ReciprocalOutMax=[]  SumDenOutMin=[]  SumDenOutMax=[]  SumNumOutMin=[]  SumNumOutMax=[]  DivideOutMin=[]  DivideOutMax=[]  UdiffTsProdOutMin=[]  UdiffTsProdOutMax=[]  NTsProdOutMin=[]  NTsProdOutMax=[]  UintegralTsProdOutMin=[]  UintegralTsProdOutMax=[]  UngainTsProdOutMin=[]  UngainTsProdOutMax=[]  ClampingZeroOutDataTypeStr=Inherit: Inherit via back propagation  ClampingZeroOutMin=[]  ClampingZeroOutMax=[]  FilterDenConstantOutDataTypeStr=Inherit: Inherit via back propagation  FilterDenConstantOutMin=[]  FilterDenConstantOutMax=[]  PCopyOutDataTypeStr=Inherit: Inherit via back propagation  PCopyOutMin=[]  PCopyOutMax=[]  NCopyOutDataTypeStr=Inherit: Inherit via back propagation  NCopyOutMin=[]  NCopyOutMax=[]  IntegratorContinuousStateAttributes=''  IntegratorStateMustResolveToSignalObject=off  IntegratorRTWStateStorageClass=Auto  FilterContinuousStateAttributes=''  FilterStateMustResolveToSignalObject=off  FilterRTWStateStorageClass=Auto  ParallelPVariant=InternalParameters  IdealPVariant=Disabled  IVariant=InternalParameters  DVariant=InternalParameters  IntegratorVariant=Continuous  SatVariant=Enabled  AWVariant=ContClampingParallel  PCopyVariant=Disabled  TRVariant=Disabled  FdbkBlocksVariant=Forward  IdealPFdbkVariant=Disabled  SatFdbkVariant=Disabled  DerivativeFilterVariant=ContFilter  NVariant=InternalParameters  NCopyVariant=Disabled  FilterICVariant=InternalICsFilter  IntegratorICVariant=InternalICs  ExternalResetVariant=Disabled  TRSumVariant=Passthrough  SumFdbkVariant=Disabled  SumVariant=Sum_PID  TsampFilterVariant=InternalTs  TsampNgainVariant=Passthrough  TsampIntegralVariant=Passthrough  ExternalSaturationOutDataTypeStr=Inherit: Same as second input
  Scope{,1..4} (5 alike) : Scope
  Sum1 : Sum  Inputs=|+-
  Switch : Switch  Criteria=u2 > Threshold  SaturateOnIntegerOverflow=off  InputSameDT=off
  Switch1 : Switch  Criteria=u2 > Threshold  SaturateOnIntegerOverflow=off  InputSameDT=off
  Ft : Outport
  Fb : Outport  Port=2
  wires:
  Gain2/1 -> Switch1/2
  Constant1/1 -> Switch1/3
  PID Controller1/1 -> Scope4/1, Scope/1, Gain/1, Switch/2, Gain2/1, Gain1/1  "y(t)"
  Constant/1 -> Switch/3
  Gain1/1 -> Switch1/1
  position_error/1 -> Scope2/1, Sum1/1
  Gain/1 -> Switch/1
  Switch/1 -> Ft1/1, Ft/1
  Switch1/1 -> Fb1/1, Fb/1
  dsafe/1 -> Scope1/1, Sum1/2
  Sum1/1 -> Scope3/1, PID Controller1/1  "e(t)"

== system Cruise_Control_system_simulation/Vehicle Dynamics1/mode_switch/thresh=0 ==
  In1 : Inport
  Action Port : ActionPort
  thresh : Outport
  wires:
  In1/1 -> thresh/1

== matlab function Cruise_Control_system_simulation/Vehicle Dynamics1/mode_switch/MATLAB Function1 ==
  data: er_sub_thresh input; Ft output; Ft1 input; Fb1 input; Ft2 input; Fb2 input; Fb output
function [Ft, Fb]= fcn(er_sub_thresh, Ft1, Fb1, Ft2, Fb2)
    Ft = 0; Fb = 0;
    if er_sub_thresh > 0
        Ft = Ft1; Fb = Fb1;
    else
        Fb = Fb2; Ft = Ft2;
    end
end

== matlab function Cruise_Control_system_simulation/Vehicle Dynamics1/mode_switch/MATLAB Function ==
  data: u input; y output
function y = fcn(u)
    y = 0;
    if (u < 0)
        y = 50;
    else
        y = 0;
    end
end

== matlab function Cruise_Control_system_simulation/Vehicle Dynamics for follower car/mode_switch/MATLAB Function ==
  data: mode input; thresh output; ethresh input
function thresh = change_thresh(mode, ethresh)
    thresh = 0;
    maxx = 10;

    if ethresh == 0 & mode < 0
        thresh = maxx;
    elseif ethresh == maxx & mode > 0
        thresh = 0;
    elseif ethresh == maxx & mode < 0
        thresh = maxx;
    else 
        thresh = 0;
    end

end

== matlab function Cruise_Control_system_simulation/Vehicle Dynamics for follower car/mode_switch/MATLAB Function1 ==
  data: mode input; Ft output; Ft1 input; Fb1 input; Ft2 input; Fb2 input; Fb output
function [Ft, Fb]= choose_mode(mode, Ft1, Fb1, Ft2, Fb2)
    Ft = 0; Fb = 0;
    if mode > 0
        Ft = Ft1; Fb = Fb1;
    else
        Fb = Fb2; Ft = Ft2;
    end
end
